simulink model "monteopt"  (Simulink 4.00)
settings: Solver=VariableStepDiscrete  SolverMode=SingleTasking  StartTime=0.0  StopTime=125  FixedStep=1  MaxStep=1  RelTol=1e-3  AbsTol=1e-6
StopFcn:
  | fovalues,povalues,standev,average
settings Model: RequirementInfo=9  Creator=pseca  LastModifiedBy=pseca  SaveTime=off  SaveOutput=off  LimitDataPoints=off  RTWTemplateMakefile=grt_vc.tmf  BlockReductionOpt=off

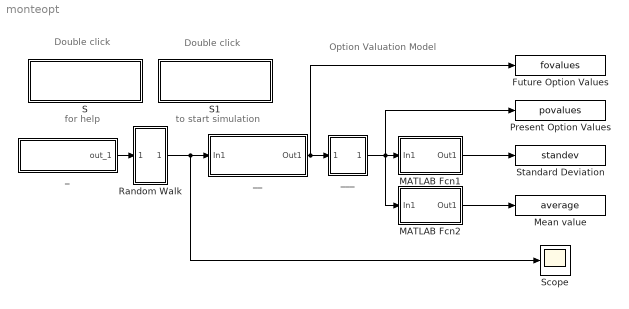
== system monteopt ==
  note: Option Valuation Model
  note: to start simulation
  note: Double click
  note: Double click
  note: for help
  Future Option Values : ToWorkspace  VariableName=fovalues  SampleTime=0  SaveFormat=Array
      settings: MaxDataPoints=1
  MATLAB Fcn1 : Subsystem
      settings: RTWFcnNameOpts=Auto  RTWFileNameOpts=Auto
      mask Type: Standard Deviation
      mask Description: Standard Deviation
      mask Help: Calculates standard deviation of option values
      mask Display: disp('STD')
  MATLAB Fcn2 : Subsystem
      settings: RTWFcnNameOpts=Auto  RTWFileNameOpts=Auto
      mask Type: Mean
      mask Description: Average Option Value
      mask Help: Calculates mean value of option prices
      mask Display: disp('Mean')
  Mean value : ToWorkspace  VariableName=average  SampleTime=0  SaveFormat=Array
      settings: MaxDataPoints=1
  Present Option Values : ToWorkspace  VariableName=povalues  SampleTime=0  SaveFormat=Array
      settings: MaxDataPoints=1
  Random Walk : Subsystem  mask(Random Walk){@1=.0185, @2=.0021, @3=5}
      mask prompts: @1 "Volatility"; @2 "Rate of Return"; @3 "# of walks"
      mask help: Random
      mask init:
      | sig = @1;ror=@2;n=@3;
      settings: RTWFcnNameOpts=Auto  RTWFileNameOpts=Auto
      mask Help: Enter the asset volality, risk-free interest rate, and the number of walks to generate.
      mask Display: plot([1 2 3 2 4 3 3.5 4 5 4.5 4.2 5])
  S : Subsystem
      settings: OpenFcn=opthelp  RTWFcnNameOpts=Auto  RTWFileNameOpts=Auto
      mask Type: Help
      mask Display: disp('Help')
  S1 : Subsystem
      settings: OpenFcn=set_param(get_param(0,'CurrentSystem'),'simulationcommand','start')  RTWFcnNameOpts=Auto  RTWFileNameOpts=Auto
      mask Type: Start
      mask Help: Double click on this block to start the simulation.
      mask Display: disp('Start')
  Scope : Scope
      settings: TickLabels=on  TimeRange=auto  YMin=60  YMax=150  SaveToWorkspace=off  SaveName=ScopeData  DataFormat=Array  LimitDataPoints=on  MaxDataPoints=5000
  Standard Deviation : ToWorkspace  VariableName=standev  SampleTime=0  SaveFormat=Array
      settings: MaxDataPoints=1
  _ : Subsystem  mask(Initialize){@1=90}
      mask prompts: @1 "Initial Value"
      mask help: Initial Asset Value
      mask init:
      | svalue = @1;
      settings: RTWFcnNameOpts=Auto  RTWFileNameOpts=Auto
      mask Help: Enter initial asset value
      mask Display: disp('Asset Value')
  __ : Subsystem  mask(Option Value ){@1=90, @2=1}
      mask prompts: @1 "Exercise Price:"; @2 "Type of option (1 for call, -1 for put):"
      mask help: Present Value of Options
      mask init:
      | strike=@1;position=@2;
      settings: RTWFcnNameOpts=Auto  RTWFileNameOpts=Auto
      mask Help: Enter option exercise price and type of option, 1 for call or -1 for put.
      mask Display: disp('Option Value')
  ___ : Subsystem  mask(Present Value ){@1=.08, @2=.5}
      mask prompts: @1 "Risk-free Interest Rate:"; @2 "Time until Maturity (years):"
      mask help: Present Value of Options
      mask init:
      | rfr=@1;tmat=@2;
      settings: RTWFcnNameOpts=Auto  RTWFileNameOpts=Auto
      mask Help: Enter risk-free interest rate and time until maturity.
      mask Display: disp('PV')
  wires:
  __/1(Out1) -> Future Option Values/1, ___/1(In1)
  Random Walk/1(out_1) -> Scope/1, __/1(In1)
  _/1(out_1) -> Random Walk/1(in_1)
  ___/1(Out1) -> MATLAB Fcn2/1(In1), Present Option Values/1, MATLAB Fcn1/1(In1)
  MATLAB Fcn2/1(Out1) -> Mean value/1
  MATLAB Fcn1/1(Out1) -> Standard Deviation/1

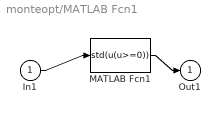
== system monteopt/MATLAB Fcn1 ==
  In1 : Inport  Port=1
  MATLAB Fcn1 : MATLABFcn  MATLABFcn=std(u(u>=0))  OutputDimensions=1  OutputSignalType=auto  Output1D=on
  Out1 : Outport  Port=1
  wires:
  In1/1 -> MATLAB Fcn1/1
  MATLAB Fcn1/1 -> Out1/1

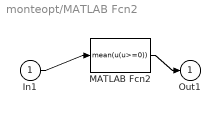
== system monteopt/MATLAB Fcn2 ==
  In1 : Inport  Port=1
  MATLAB Fcn2 : MATLABFcn  MATLABFcn=mean(u(u>=0))  OutputDimensions=1  OutputSignalType=auto  Output1D=on
  Out1 : Outport  Port=1  InitialOutput=0
  wires:
  In1/1 -> MATLAB Fcn2/1
  MATLAB Fcn2/1 -> Out1/1

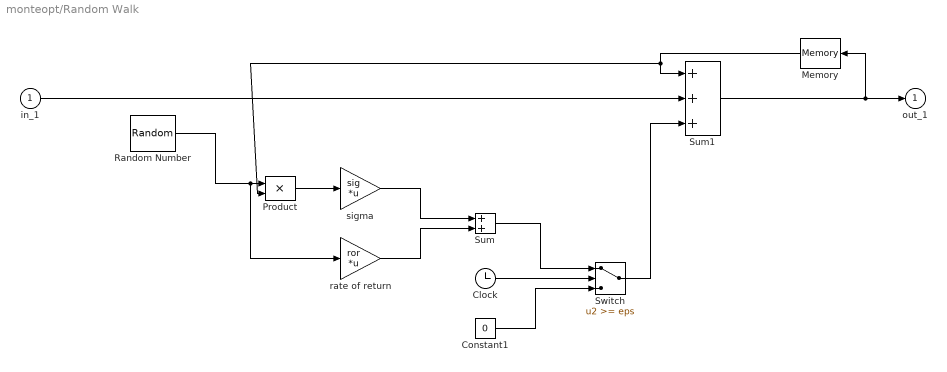
== system monteopt/Random Walk ==
  in_1 : Inport  Port=1
  Clock : Clock
      settings: DisplayTime=off  Decimation=10
  Constant1 : Constant  Value=0
  Memory : Memory  Orientation=left  X0=0  InheritSampleTime=off
  Product : Product  Inputs=2  Multiplication=Element-wise(.*)  SaturateOnIntegerOverflow=on
  Random Number : RandomNumber  Mean=0  Variance=1  Seed=123456*rand(1,n)  SampleTime=0
  Sum : Sum  Inputs=++  SaturateOnIntegerOverflow=on
  Sum1 : Sum  Inputs=+++  SaturateOnIntegerOverflow=on
  Switch : Switch  Threshold=eps
  rate of return : Gain  Gain=ror  Multiplication=Matrix(K*u)  SaturateOnIntegerOverflow=on
  sigma : Gain  Gain=sig  Multiplication=Matrix(K*u)  SaturateOnIntegerOverflow=on
  out_1 : Outport  Port=1  InitialOutput=0
  wires:
  Random Number/1 -> rate of return/1, Product/1
  Memory/1 -> Product/2, Sum1/1
  Sum1/1 -> out_1/1, Memory/1
  in_1/1 -> Sum1/2
  Switch/1 -> Sum1/3
  Product/1 -> sigma/1
  Sum/1 -> Switch/1
  Constant1/1 -> Switch/3
  Clock/1 -> Switch/2
  rate of return/1 -> Sum/2
  sigma/1 -> Sum/1

== system monteopt/S ==

== system monteopt/S1 ==

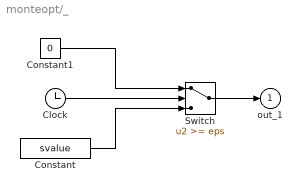
== system monteopt/_ ==
  Clock : Clock
      settings: DisplayTime=off  Decimation=10
  Constant : Constant  Value=svalue
  Constant1 : Constant  Value=0
  Switch : Switch  Threshold=eps
  out_1 : Outport  Port=1  InitialOutput=0
  wires:
  Switch/1 -> out_1/1
  Constant/1 -> Switch/3
  Clock/1 -> Switch/2
  Constant1/1 -> Switch/1

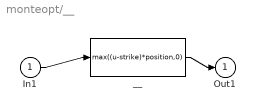
== system monteopt/__ ==
  In1 : Inport  Port=1
  __ : MATLABFcn  MATLABFcn=max((u-strike)*position,0)  OutputDimensions=-1  OutputSignalType=auto  Output1D=on
  Out1 : Outport  Port=1  InitialOutput=0
  wires:
  In1/1 -> __/1
  __/1 -> Out1/1

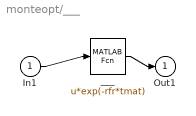
== system monteopt/___ ==
  In1 : Inport  Port=1
  ___ : MATLABFcn  MATLABFcn=u*exp(-rfr*tmat)  OutputDimensions=-1  OutputSignalType=auto  Output1D=on
  Out1 : Outport  Port=1  InitialOutput=0
  wires:
  In1/1 -> ___/1
  ___/1 -> Out1/1
